simulink model "Hopper_6dof_nonlinear_model_openLoop"  (R2025b)
settings: Solver=VariableStepAuto  StartTime=0.0  StopTime=10  RelTol=1e-3
model workspace (MAT data in the model file):
  op_trim2 = opcond.OperatingReport
  op_trim2.Outputs_ = opcond.OutputReport
  op_trim2.Outputs_.yspec_ = 0
  op_trim2.Outputs_.Block_ = 'hopper_6dof_nonlinear_model/Z'
  op_trim2.Outputs_.PortWidth_ = 1
  op_trim2.Outputs_.PortNumber_ = NaN
  op_trim2.Outputs_.y_ = 50
  op_trim2.Outputs_.Known_ = 0
  op_trim2.Outputs_.Min_ = -Inf
  op_trim2.Outputs_.Max_ = Inf
  op_trim2.TerminationString_ = 'Operating point specifications were successfully met.'
  op_trim2.OptimizationOutput_.iterations = 2
  op_trim2.OptimizationOutput_.funcCount = 8
  op_trim2.OptimizationOutput_.lssteplength = 1
  op_trim2.OptimizationOutput_.stepsize = 0.000935555393881
  op_trim2.OptimizationOutput_.algorithm = 'active-set'
  op_trim2.OptimizationOutput_.firstorderopt = 8.9494364321e-10
  op_trim2.OptimizationOutput_.constrviolation = 2.72848410532e-14
  op_trim2.OptimizationOutput_.message = 'Local minimum found that satisfies the constraints.
    | 
    | Optimization completed because the objective function is non-decreasing in 
    | feasible directions, to within the value of the optimality tolerance,
    | and constraints are satisfied to within the  value of the constraint tolerance.
    | 
    | <stopping criteria details>
    | 
    | Optimization completed: The first-order optimality measure, 8.949436e-10, is less
    | than options.OptimalityTolerance = 1.000000e-06, and the maximum constraint violation,
    | 2.728484e-14,is less than options.ConstraintTolerance = 1.000000e-06.'
  op_trim2.OptimizationOutput_.bestfeasible.x = 981
  op_trim2.OptimizationOutput_.bestfeasible.fval = 0
  op_trim2.OptimizationOutput_.bestfeasible.constrviolation = 2.72848410532e-14
  op_trim2.OptimizationOutput_.bestfeasible.firstorderopt = 8.9494364321e-10
  op_trim2.OptimizationOutput_.progress = {'<font face="monospaced"; size=3><BR>', 'Optimizing to solve for all desired dx/dt=0, x(k+1)-x(k)=0, and y=ydes.<BR>', ' <BR>', '(Maximum Error)  Block<BR>', ' ---------------------------------------------------------<BR>', '(9.81000e+00) hopper_6dof_nonlinear_model/Integrator (X Y Z ,u v w, P Q R, q0 q1 q2 q3) <BR>', '(9.35555e-06) hopper_6dof_nonlinear_model/Integrator (X Y Z ,u v w, P Q R, q0 q1 q2 q3) <BR>', '(2.72848e-14) hopper_6dof_nonlinear_model/Integrator (X Y Z ,u v w, P Q R, q0 q1 q2 q3) <BR>', '(2.72848e-14) hopper_6dof_nonlinear_model/Integrator (X Y Z ,u v w, P Q R, q0 q1 q2 q3) <BR>', ' <BR>', 'Operating point specifications were successfully met.<BR>'}
  op_trim2.Model_ = 'hopper_6dof_nonlinear_model'
  op_trim2.States_ = opcond.StateReport
  op_trim2.States_.dx_ = [0; 0; 0; 2.72848410532e-14; 0; 0; 0; 0; 0; 0; 0; 0; 0]
  op_trim2.States_.Nx_ = 13
  op_trim2.States_.Block_ = 'hopper_6dof_nonlinear_model/Integrator (X Y Z ,u v w, P Q R, q0 q1 q2 q3) '
  op_trim2.States_.x_ = [0; 0; 50; 0; 0; 0; 0; 0; 0; 0.707106781187; 0; 0.707106781187; 0]
  op_trim2.States_.SteadyState_ = [1; 1; 0; 1; 1; 1; 1; 1; 1; 1; 1; 1; 1]
  op_trim2.States_.dxMin_ = [-Inf; -Inf; -Inf; -Inf; -Inf; -Inf; -Inf; -Inf; -Inf; -Inf; -Inf; -Inf; -Inf]
  op_trim2.States_.dxMax_ = [Inf; Inf; Inf; Inf; Inf; Inf; Inf; Inf; Inf; Inf; Inf; Inf; Inf]
  op_trim2.States_.Known_ = [1; 1; 1; 1; 1; 1; 1; 1; 1; 1; 1; 1; 1]
  op_trim2.States_.Min_ = [-Inf; -Inf; -Inf; -Inf; -Inf; -Inf; -Inf; -Inf; -Inf; -Inf; -Inf; -Inf; -Inf]
  op_trim2.States_.Max_ = [Inf; Inf; Inf; Inf; Inf; Inf; Inf; Inf; Inf; Inf; Inf; Inf; Inf]
  op_trim2.Inputs_(1) = opcond.InputReport
  op_trim2.Inputs_(1).Block_ = 'hopper_6dof_nonlinear_model/Thrust'
  op_trim2.Inputs_(1).PortWidth_ = 1
  op_trim2.Inputs_(1).PortDimensions_ = [1 1]
  op_trim2.Inputs_(1).u_ = 981
  op_trim2.Inputs_(1).Known_ = 0
  op_trim2.Inputs_(1).Min_ = -Inf
  op_trim2.Inputs_(1).Max_ = Inf
  op_trim2.Inputs_(2) = opcond.InputReport
  op_trim2.Inputs_(2).Block_ = 'hopper_6dof_nonlinear_model/delta_p'
  op_trim2.Inputs_(2).PortWidth_ = 1
  op_trim2.Inputs_(2).PortDimensions_ = [1 1]
  op_trim2.Inputs_(2).Known_ = 1
  op_trim2.Inputs_(2).Min_ = -Inf
  op_trim2.Inputs_(2).Max_ = Inf
  op_trim2.Inputs_(3) = opcond.InputReport
  op_trim2.Inputs_(3).Block_ = 'hopper_6dof_nonlinear_model/delta_y'
  op_trim2.Inputs_(3).PortWidth_ = 1
  op_trim2.Inputs_(3).PortDimensions_ = [1 1]
  op_trim2.Inputs_(3).Known_ = 1
  op_trim2.Inputs_(3).Min_ = -Inf
  op_trim2.Inputs_(3).Max_ = Inf
undefined symbols (not defined in the file or in its folder): x0
libraries: aerolibanim x1, sharedtransform x1
settings Model: Creator=vip  LastModifiedBy=vip
settings DataIOCC: ExternalInput=getinputstruct(op_trim1)  InitialState=getstatestruct(op_trim1)

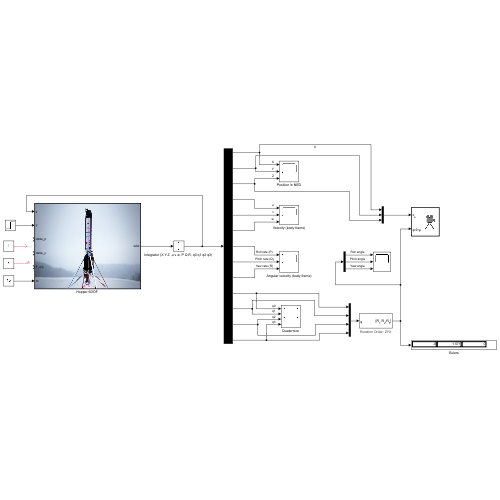
[thumbnail: Simulink's stored preview of the top-level diagram]
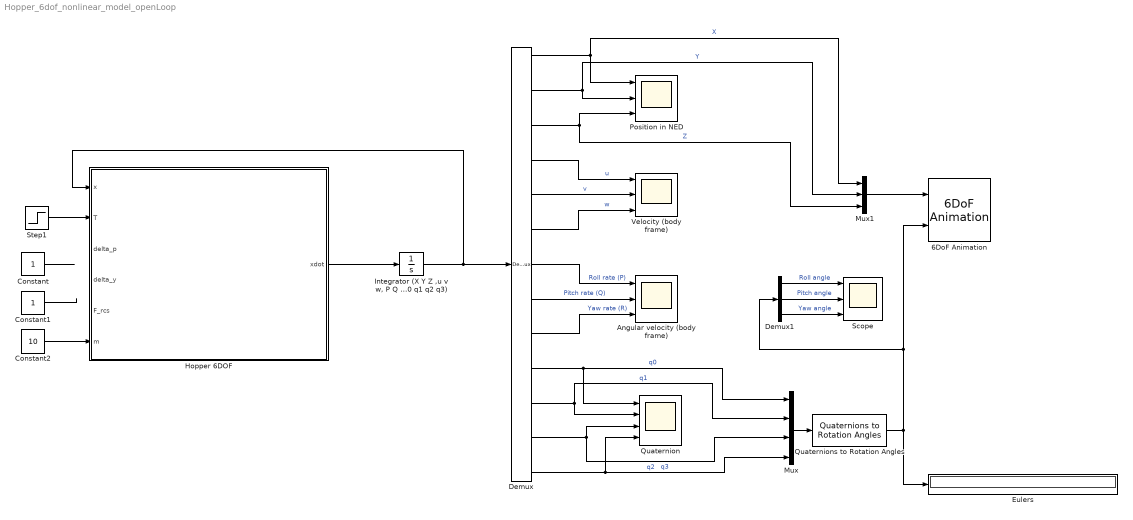
== system Hopper_6dof_nonlinear_model_openLoop ==
  6DoF Animation : aerolibanim/6DoF Animation  u1=[0 5000 -10 10 -10 10]  u2=0.1  u3=25  u4=[4000 0 -5000]  u5=Fly alongside  u6=[20 50 -10]  u7=45  u8=on
  Angular velocity (body frame) : Scope  NumInputPorts=3
      settings: ActiveDisplayYMinimum=-1  ActiveDisplayYMaximum=1  DataLoggingVariableName=ScopeData2
  Constant : Constant
  Constant1 : Constant
  Constant2 : Constant  Value=10
  Demux : Demux  Outputs=13
  Demux1 : Demux  Outputs=3
  Eulers : Display
  "Hopper 6DOF " : MATLAB Function  TreatAsAtomicUnit=on
  "Integrator (X Y Z ,u v w, P Q R, q0 q1 q2 q3) " : Integrator  InitialCondition=x0
  Mux : Mux
  Mux1 : Mux  Inputs=3
  Position in NED : Scope  NumInputPorts=3
      settings: ActiveDisplayYMinimum=-27572.669229824489  ActiveDisplayYMaximum=3063.6299144249429
  Quaternion : Scope  NumInputPorts=4
      settings: ActiveDisplayYMinimum=-0.88387  ActiveDisplayYMaximum=0.88387
  Quaternions to Rotation Angles : sharedtransform/Quaternions to Rotation Angles  rotationOrder=ZYX  aMode=aMode
  Scope : Scope  NumInputPorts=3
      settings: ActiveDisplayYMinimum=-0.19635  ActiveDisplayYMaximum=1.76715
  Step1 : Step  Time=0  After=5000  SampleTime=0
  Velocity (body frame) : Scope  NumInputPorts=3
      settings: ActiveDisplayYMinimum=-612.73773519475014  ActiveDisplayYMaximum=5514.6396167527528
  wires:
  "Integrator (X Y Z ,u v w, P Q R, q0 q1 q2 q3) "/1 -> "Hopper 6DOF "/1(x), Demux/1
  Demux/5 -> Velocity (body frame)/2  "v"
  Demux/4 -> Velocity (body frame)/1  "u"
  Demux/6 -> Velocity (body frame)/3  "w"
  Demux/2 -> Position in NED/2, Mux1/2  "Y"
  Demux/1 -> Position in NED/1, Mux1/1  "X"
  Demux/3 -> Mux1/3, Position in NED/3  "Z"
  Demux/7 -> Angular velocity (body frame)/1  "Roll rate (P)"
  Demux/8 -> Angular velocity (body frame)/2  "Pitch rate (Q)"
  Demux/9 -> Angular velocity (body frame)/3  "Yaw rate (R)"
  Demux/10 -> Mux/1, Quaternion/1  "q0"
  Demux/11 -> Mux/2, Quaternion/2  "q1"
  Demux/12 -> Quaternion/3, Mux/3  "q2"
  Demux/13 -> Mux/4, Quaternion/4  "q3"
  "Hopper 6DOF "/1(xdot) -> "Integrator (X Y Z ,u v w, P Q R, q0 q1 q2 q3) "/1
  Mux/1 -> Quaternions to Rotation Angles/1
  Demux1/1 -> Scope/1  "Roll angle"
  Demux1/2 -> Scope/2  "Pitch angle"
  Demux1/3 -> Scope/3  "Yaw angle"
  Quaternions to Rotation Angles/1 -> Eulers/1, 6DoF Animation/2, Demux1/1
  Mux1/1 -> 6DoF Animation/1
  Constant/1 -> ?
  Constant1/1 -> ?
  Constant2/1 -> "Hopper 6DOF "/6(m)
  Step1/1 -> "Hopper 6DOF "/2(T)

== matlab function Hopper_6dof_nonlinear_model_openLoop/Hopper 6DOF  ==
  data: x input; xdot output; T input; delta_p input; delta_y input; F_rcs input; m input
function xdot= hopper6dof2(x, T, delta_p, delta_y, F_rcs, m)
% 6-DOF hopper dynamics with time-varying mass & inertia
%% ==== STATES ====
X  = x(1); 
Y  = x(2); 
Z  = x(3);
u  = x(4);
v  = x(5);
w  = x(6);
P  = x(7); 
Q  = x(8);
R  = x(9);
q0 = x(10); 
q1 = x(11); 
q2 = x(12); 
q3 = x(13);

%% ==== CONSTANTS ====
m0  = 100;          % initial mass [kg]
mdot = 0.5;         % mass burn rate [kg/s]

D_m = 0.25;
r_m = D_m / 2;
L_m = 4;
g   = 9.81;

%% ==== INERTIA (scaled with mass, JUST initially) ====
Ix0 = 0.5 * m0 * r_m^2;
Iy0 = (1/12) * m0 * (3*r_m^2 + L_m^2);
Iz0 = Iy0;

Ix = Ix0 * (m / m0);
Iy = Iy0 * (m / m0);
Iz = Iz0 * (m / m0);
Ixz = 0;

%% ==== ROTATION MATRIX ====
Rbody2NED = [ ...
 q0^2+q1^2-q2^2-q3^2, 2*(q1*q2-q0*q3),   2*(q1*q3+q0*q2);
 2*(q1*q2+q0*q3),   q0^2-q1^2+q2^2-q3^2, 2*(q2*q3-q0*q1);
 2*(q1*q3-q0*q2),   2*(q2*q3+q0*q1),   q0^2-q1^2-q2^2+q3^2 ];

%% ==== FORCES ====
Fx_T =  T * cosd(delta_p) * cosd(delta_y);
Fy_T = -T * cosd(delta_p) * sind(delta_y);
Fz_T = -T * sind(delta_p);

F_g_body = Rbody2NED.' * [0; 0; m*g];

Fx = Fx_T + F_g_body(1);
Fy = Fy_T + F_g_body(2);
Fz = Fz_T + F_g_body(3);

udot = Fx/m - Q*w + R*v;
vdot = Fy/m - R*u + P*w;
wdot = Fz/m - P*v + Q*u;

%% ==== MOMENTS ====
d = 1;   
r = [-d; 0; 0]; % In body frame x axes is along the centerline 
F_T = [Fx_T; Fy_T; Fz_T];
M_TVC = cross(r, F_T);

n_rcs = 2;
L = M_TVC(1) + r_m * F_rcs * n_rcs; % Roll moment 
M = M_TVC(2);                                     % Pitch moment 
N = M_TVC(3);                                       % Yaw moment 


% Rotational EOM
% p_dot
pdot = ( Iz*L + Ixz*N ...
       + (Ixz^2 - Iz*Iy)*Q*R ...
       + Ixz*(Ix - Iy)*P*Q ) ...
       / (Ix*Iz - Ixz^2);

% q_dot
qdot = ( M ...
       + (Iz - Ix)*P*R ...
       - Ixz*(P^2 - R^2) ) / Iy;

% r_dot
rdot = ( Ix*N + Ixz*L ...
       + (Ixz^2 - Ix*Iy)*P*Q ...
       + Ixz*(Iy - Iz)*Q*R ) ...
       / (Ix*Iz - Ixz^2);

%% ==== QUATERNION KINEMATICS ====
q0dot = -0.5*(q1*P + q2*Q + q3*R);
q1dot =  0.5*(q0*P + q2*R - q3*Q);
q2dot =  0.5*(q0*Q + q3*P - q1*R);
q3dot =  0.5*(q0*R + q1*Q - q2*P);

%% ==== POSITION KINEMATICS ====
pos_dot = Rbody2NED * [u; v; w];

%% ==== PACK ALL STATES====
xdot = [
 pos_dot;
 udot; vdot; wdot;
 pdot; qdot; rdot;
 q0dot; q1dot; q2dot; q3dot ];

end
